simulink model "leaderAppl"  (R2022a)
settings: Solver=ode1  StartTime=0.0  StopTime=Inf  FixedStep=0.001  RelTol=1e-3
PreLoadFcn:
  | % 64-bit float
  | TurnSignalLeverValue = Simulink.Parameter;
  | TurnSignalLeverValue.StorageClass = 'ExportedGlobal';
  | TurnSignalLeverValue.DataType = 'double'
  | TurnSignalLeverValue.Value = 0.0
  | 
  | % 64-bit float
  | WarningLightSwitchValue= Simulink.Parameter;
  | WarningLightSwitchValue.StorageClass = 'ExportedGlobal';
  | WarningLightSwitchValue.DataType = 'double'
  | WarningLightSwitchValue.Value = 0.0
  | 
  | % 64-bit float
  | BatteryVoltageValue = Simulink.Parameter;
  | BatteryVoltageValue.StorageClass = 'ExportedGlobal';
  | BatteryVoltageValue.DataType = 'double'
  | BatteryVoltageValue.Value = 12.5
  | 
  | % 64-bit float
  | SyncValue = Simulink.Parameter;
  | SyncValue.StorageClass = 'ExportedGlobal';
  | SyncValue.DataType = 'double'
  | SyncValue.Value = 0.0
  | 
  | % 64-bit float
  | WarningLightIndicator = Simulink.Signal;
  | WarningLightIndicator.StorageClass = 'ExportedGlobal';
  | 
  | % 64-bit float
  | FrontLightEcuTurnSignalLeft = Simulink.Signal;
  | FrontLightEcuTurnSignalLeft.StorageClass = 'ExportedGlobal';
  | 
  | % 64-bit float
  | FrontLightEcuTurnSignalRight = Simulink.Signal;
  | FrontLightEcuTurnSignalRight.StorageClass = 'ExportedGlobal';
  | 
  | % 64-bit float
  | RearLightEcuTurnSignalLeft = Simulink.Signal;
  | RearLightEcuTurnSignalLeft.StorageClass = 'ExportedGlobal';
  | 
  | % 64-bit float
  | RearLightEcuTurnSignalRight = Simulink.Signal;
  | RearLightEcuTurnSignalRight.StorageClass = 'ExportedGlobal';
PostLoadFcn:
  | , if any(exist('dsrtsu_mdlpostloadfcn', 'file') ~= 0), dsrtsu_mdlpostloadfcn('Execute', bdroot); end,
  | 
  | % Begin Version: 1.0
  | if(3 == exist('DSWatchDog')), DSWatchDog('OpenModel', get_param(bdroot(gcs),'filename')); end; assignin('base', sprintf('DS_%s_STATE', upper(bdroot(gcs))), 0);
  | % End Version: 1.0
InitFcn:
  | , if any(exist('rtifpga_mdlclblib', 'file') ~= 0), rtifpga_mdlclblib('Init', bdroot); end,
  | , if any(exist('dsmpb_private', 'file') ~= 0), dsmpb_private('dsmpb_mdlclblib', 'Init', bdroot); end,
StartFcn:
  | % Begin Version: 1.0
  | if(3 == exist('DSWatchDog')), DSWatchDog('StartModel', get_param(bdroot(gcs),'filename')); end; assignin('base', sprintf('DS_%s_STATE', upper(bdroot(gcs))), 2);
  | % End Version: 1.0
StopFcn:
  | % Begin Version: 1.0
  | if(3 == exist('DSWatchDog')), DSWatchDog('StopModel', get_param(bdroot(gcs),'filename')); end; assignin('base', sprintf('DS_%s_STATE', upper(bdroot(gcs))), 0);
  | % End Version: 1.0
libraries: simulink x2, simulink_extras x2
PreSaveFcn:
  | , if any(exist('dsmpb_private', 'file') ~= 0), dsmpb_private('dsmpb_mdlclblib', 'PreSave', bdroot); end,
  | 
  | % Begin Version: 1.0
  | OldName = get_param(bdroot(gcs), 'Tag'); NewName = get_param(bdroot(gcs), 'filename'); if (~strcmp(OldName, NewName)), if(3 == exist('DSWatchDog')), DSWatchDog('CloseModel', OldName); DSWatchDog('OpenModel', NewName); end; set_param(bdroot(gcs), 'Tag', NewName); end; try, evalin('base', 'clear OldName NewName'); catch, disp('Error during execution of PreSaveFcn callback'); end;
  | % End Version: 1.0
PostSaveFcn:
  | % Begin Version: 1.0
  | if(3 == exist('DSWatchDog')), DSWatchDog('SaveModel', get_param(bdroot(gcs),'filename')); end;
  | % End Version: 1.0
CloseFcn:
  | , if any(exist('dsmpb_private', 'file') ~= 0), dsmpb_private('dsmpb_mdlclblib', 'Close', bdroot); end,
  | % Begin Version: 1.0
  | if(3 == exist('DSWatchDog')), DSWatchDog('CloseModel', get_param(bdroot(gcs),'filename')); end; try, DS_STATE_NAME = sprintf('DS_%s_STATE', upper(bdroot(gcs))); evalin('base', 'clear(DS_STATE_NAME)'); evalin('base', 'clear DS_STATE_NAME'); catch, disp('Error during execution of CloseFcn callback'); end;
  | % End Version: 1.0
settings Model: Tag=C:\Users\dSPACE GmbH\Documents\dSPACE\Real-Time Testing\2023-B\SampleExperiments\TurnSignal_VEOSVECUMC\TurnSignal_VEOSVECUMC\Models\masterAppl.slx  RTICANMMDATA=struct('GeneralSetupData',struct('modelroot',['C:\Users\Admin\Documents\dSPACE\Real-Time Testing\3.2\SampleExperiments\TurnSignal_VEOSMC\Model'],'generalsettings',struct('filesettings',struct('destfolder',struct('Name','RTICANMM_FILES','Check',1),'buildfolder',struct('Name','.','Check',1),'AbsDestfolder',struct('Name',['C:\Users\Admin\Documents\dSPACE\Real-Time Testing\3.2\SampleExperiments\TurnSignal_VEOSMC\Model\RTICANMM_FILES']),'AbsBuildfolder',struct('Name',['C:\Users\Admin\Documents\dSPACE\Real-Time Testing\3.2\SampleExperiments\TurnSignal_VEOSMC\Model']))),'options',struct('addpaths',1,'rmpaths',1,'addtrcexclusion',logical(1),'cannavigator',struct('checkmonitoring',0),'show_usrtrc',0,'use_usrtrc',0),'advanced',struct('options',ones(1,100)),'MPSetup',{{}},'modelname','masterAppl','block','masterAppl'))  RTILINMMDATA=struct('GeneralSetupData',[])  DSRTSU_INTERNAL_RTI_VER=620  DSRTSU_INTERNAL_RTI_TYPE=rti1202  DSRTSU_INTERNAL_RTIFPGA=200  DSRTSU_INTERNAL_RTISTBM_VER=23.2  ModifiedByFormat=dSPACE GmbH  ExtModeTrigMode=oneshot  ExtModeArmWhenConnect=off  Creator=dSPACE GmbH  LastModifiedBy=dSPACE GmbH
settings SolverCC: AlgebraicLoopSolver=TrustRegion
settings DataIOCC: LimitDataPoints=on  SaveFormat=Structure  SignalLoggingSaveFormat=ModelDataLogs  ReturnWorkspaceOutputs=off
settings OptimizationCC: BlockReduction=off  ConditionallyExecuteInputs=off  OptimizeBlockIOStorage=off  BufferReuse=off  GlobalBufferReuse=off  ExpressionFolding=off  ExpressionDepthLimit=2147483647  LocalBlockOutputs=off  InitFltsAndDblsToZero=on  LifeSpan=inf
settings DebuggingCC: SaveWithParameterizedLinksMsg=none  UnderspecifiedInitializationDetection=Classic  MergeDetectMultiDrivingBlocksExec=none  SignalResolutionControl=TryResolveAllWithWarning  MultiTaskDSMMsg=warning  MultiTaskCondExecSysMsg=none  MultiTaskRateTransMsg=warning  TasksWithSamePriorityMsg=none  FcnCallInpInsideContextMsg=warning  UnconnectedInputMsg=warning  UnconnectedOutputMsg=warning  UnconnectedLineMsg=warning  AllowSymbolicDim=off  StateNameClashWarn=warning  SFUnexpectedBacktrackingDiag=warning  SFNoUnconditionalDefaultTransitionDiag=warning  SFExecutionAtInitializationDiag=none  SFMachineParentedDataDiag=warning  ArithmeticOperatorsInVariantConditions=warning
settings HardwareCC: ProdBitPerLong=64  ProdLargestAtomicInteger=Integer  ProdWordSize=32  ProdHWDeviceType=Custom Processor->Custom  TargetIntDivRoundTo=Zero  TargetEndianess=LittleEndian  TargetHWDeviceType=Generic->Custom
settings ModelReferenceCC: PropagateSignalLabelsOutOfModel=off
settings SFSimCC: SimUseLocalCustomCode=off  CustomCodeUndefinedFunction=UseInterfaceOnly
settings RTWCC: Description=dSPACE Run-Time Target  SystemTargetFile=dsrt.tlc  GenCodeOnly=on  MakeCommand=make_dsrt  TemplateMakefile=dsrt_default_tmf  RTWVerbose=off  RTWUseLocalCustomCode=off
settings CodeAppCC: StateflowObjectComments=on
settings STFCustomTargetCC: ParMdlRefBuildCompliant=on  GRTInterface=off  SystemTargetFile=dsrt.tlc
settings GRTTargetCC: TargetLangStandard=C89/C90 (ANSI)  CompOptLevelCompliant=off  ConcurrentExecutionCompliant=off  CombineOutputUpdateFcns=off  MatFileLogging=off  CPPClassGenCompliant=off  UseToolchainInfoCompliant=off  GenerateASAP2=on
settings ConfigComp: CovMetricSettings=dw  CovSaveCumulativeToWorkspaceVar=on  CovSaveSingleToWorkspaceVar=on  CovExternalEMLEnable=off  CovSFcnEnable=off

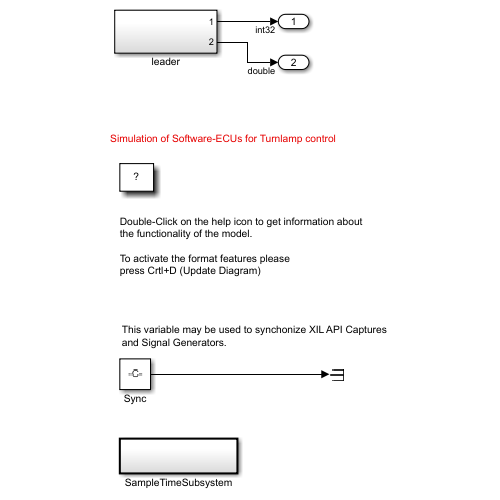
[thumbnail: Simulink's stored preview of the top-level diagram]
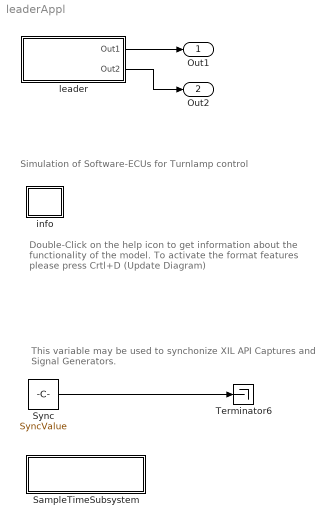
== system leaderAppl ==
  note: Simulation of Software-ECUs for Turnlamp control
  note: Double-Click on the help icon to get information about
      | the functionality of the model.
      |
      | To activate the format features please
      | press Crtl+D (Update Diagram)
  note: This variable may be used to synchonize XIL API Captures
      | and Signal Generators.
  SampleTimeSubsystem : Subsystem  TreatAsAtomicUnit=on  SystemSampleTime=0.01
  Sync : Constant  Value=SyncValue
  Terminator6 : Terminator
  info : Subsystem
      mask Display: disp('?')
  leader : Subsystem
  Out1 : Outport  OutDataTypeStr=int32  PortDimensions=1
  Out2 : Outport  Port=2  OutDataTypeStr=double  PortDimensions=1
  wires:
  leader/1(Out1) -> Out1/1
  leader/2(Out2) -> Out2/1
  Sync/1 -> Terminator6/1

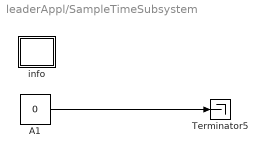
== system leaderAppl/SampleTimeSubsystem ==
  A1 : Constant  Value=0
  Terminator5 : Terminator
  info : Subsystem
      mask Display: disp('?')
  wires:
  A1/1 -> Terminator5/1

== system leaderAppl/info ==
  note: .
  note: This model simulates the behaviour of three ECUs for controlling TurnSignals,
      | dependent on a TurnSignalLever and a WarningLightSwitch
  note: Aim of this demo: to show possibilities of different ECU test procedures
  note: To control this model, use the corresponding ControlDesk experiment:
      | - Set TurnSignalLever to Left, Right or Off
      | - Switch WarningLight Switch to Off or On
      | - Change the Battery voltage: below a certain voltage level, some (simulated) malfunctions may occur
      |    - <= 7.2V, the ECUs will collapse completely
      |    - <= 8.2 V (dependent on voltage, more effect with lower voltage), simulated receiver in front and rear ECU become unstable,
      |      thus the timing of the generated TurnSignal will be disturbed

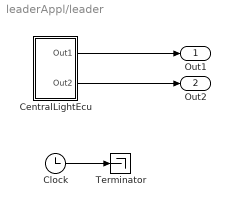
== system leaderAppl/leader ==
  CentralLightEcu : Subsystem
  Clock : Clock
  Terminator : Terminator
  Out1 : Outport
  Out2 : Outport  Port=2
  wires:
  CentralLightEcu/1(Out1) -> Out1/1
  CentralLightEcu/2(Out2) -> Out2/1
  Clock/1 -> Terminator/1

== system leaderAppl/SampleTimeSubsystem/info ==
  note: .
  note: This subsystems realizes a new sampling period for measurements. It is configured with a step size of 10 ms.

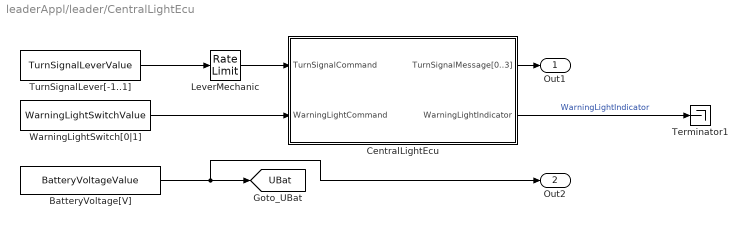
== system leaderAppl/leader/CentralLightEcu ==
  BatteryVoltage[V] : Constant  Value=BatteryVoltageValue
  CentralLightEcu : Subsystem
  LeverMechanic : RateLimiter  RisingSlewLimit=25  FallingSlewLimit=-25
  Terminator1 : Terminator
  TurnSignalLever[-1..1] : Constant  Value=TurnSignalLeverValue
  WarningLightSwitch[0|1] : Constant  Value=WarningLightSwitchValue
  Out1 : Outport
  Out2 : Outport  Port=2
  tag scope: UBat=global
  wires:
  CentralLightEcu/1(TurnSignalMessage[0..3]) -> Out1/1
  BatteryVoltage[V]/1 -> Out2/1, [UBat]
  CentralLightEcu/2(WarningLightIndicator) -> Terminator1/1  "WarningLightIndicator"
  WarningLightSwitch[0|1]/1 -> CentralLightEcu/2(WarningLightCommand)
  LeverMechanic/1 -> CentralLightEcu/1(TurnSignalCommand)
  TurnSignalLever[-1..1]/1 -> LeverMechanic/1

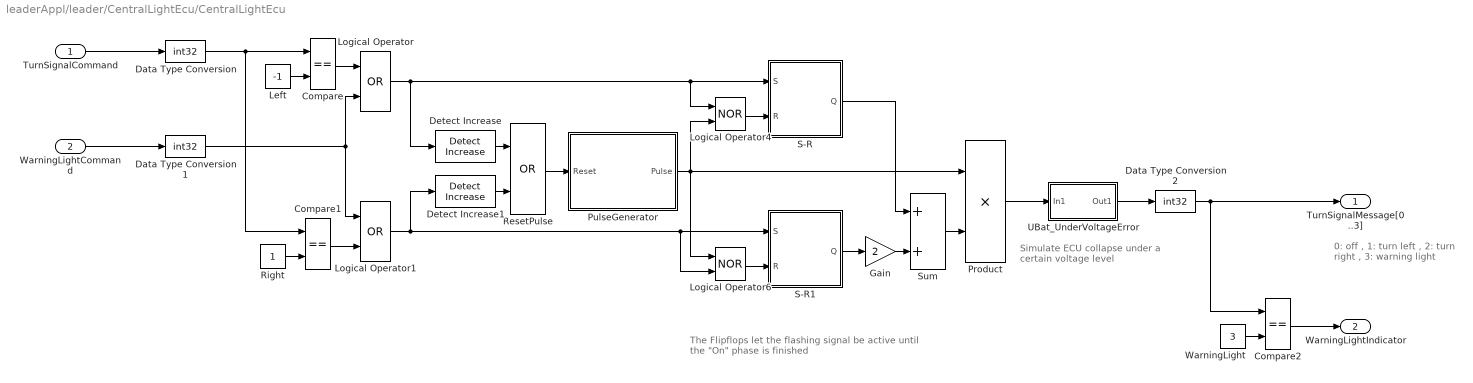
== system leaderAppl/leader/CentralLightEcu/CentralLightEcu ==
  note: The Flipflops let the flashing signal be active until
      | the "On" phase is finished
  note: Simulate ECU collapse
      | under a certain voltage level
  note: 0: off               ,
      | 1: turn left       ,
      | 2: turn right     ,
      | 3: warning light
  TurnSignalCommand : Inport
  WarningLightCommand : Inport  Port=2
  Compare : RelationalOperator  Operator===  OutDataTypeStr=uint(8)  ZeroCross=off
  Compare1 : RelationalOperator  Operator===  OutDataTypeStr=uint(8)  ZeroCross=off
  Compare2 : RelationalOperator  Operator===  OutDataTypeStr=uint(8)  ZeroCross=off
  Data Type Conversion : DataTypeConversion  OutDataTypeStr=int32  SaturateOnIntegerOverflow=off
  Data Type Conversion1 : DataTypeConversion  OutDataTypeStr=int32  SaturateOnIntegerOverflow=off
  Data Type Conversion2 : DataTypeConversion  OutDataTypeStr=int32  SaturateOnIntegerOverflow=off
  Detect Increase : simulink/Logic and Bit Operations/Detect Increase  vinit=0.0  OutDataTypeStr=boolean
  Detect Increase1 : simulink/Logic and Bit Operations/Detect Increase  vinit=0.0  OutDataTypeStr=boolean
  Gain : Gain  Gain=2
  Left : Constant  Value=-1  OutDataTypeStr=Inherit: Inherit via back propagation
  Logical Operator : Logic  Operator=OR  AllPortsSameDT=off  OutDataTypeStr=uint(8)
  Logical Operator1 : Logic  Operator=OR  AllPortsSameDT=off  OutDataTypeStr=uint(8)
  Logical Operator4 : Logic  Operator=NOR  AllPortsSameDT=off  OutDataTypeStr=uint(8)
  Logical Operator6 : Logic  Operator=NOR  AllPortsSameDT=off  OutDataTypeStr=uint(8)
  Product : Product  RndMeth=Zero
  PulseGenerator : Subsystem
  ResetPulse : Logic  Operator=OR  AllPortsSameDT=off  OutDataTypeStr=uint(8)
  Right : Constant  OutDataTypeStr=Inherit: Inherit via back propagation
  S-R : Subsystem
  S-R1 : Subsystem
  Sum : Sum
  UBat_UnderVoltageError : Subsystem
  WarningLight : Constant  Value=3  OutDataTypeStr=Inherit: Inherit via back propagation
  TurnSignalMessage[0..3] : Outport  OutDataTypeStr=int32
  WarningLightIndicator : Outport  Port=2
  wires:
  WarningLight/1 -> Compare2/2
  Right/1 -> Compare1/2
  Left/1 -> Compare/2
  Data Type Conversion2/1 -> Compare2/1, TurnSignalMessage[0..3]/1
  UBat_UnderVoltageError/1(Out1) -> Data Type Conversion2/1
  S-R/1(Q) -> Sum/1
  S-R1/1(Q) -> Gain/1
  Sum/1 -> Product/2
  PulseGenerator/1(Pulse) -> Product/1, Logical Operator6/1, Logical Operator4/2
  ResetPulse/1 -> PulseGenerator/1(Reset)
  Detect Increase1/1 -> ResetPulse/2
  Detect Increase/1 -> ResetPulse/1
  Logical Operator1/1 -> S-R1/1(S), Logical Operator6/2, Detect Increase1/1
  Logical Operator6/1 -> S-R1/2(R)
  Logical Operator4/1 -> S-R/2(R)
  Logical Operator/1 -> Detect Increase/1, S-R/1(S), Logical Operator4/1
  Compare2/1 -> WarningLightIndicator/1
  WarningLightCommand/1 -> Data Type Conversion1/1
  Product/1 -> UBat_UnderVoltageError/1(In1)
  TurnSignalCommand/1 -> Data Type Conversion/1
  Gain/1 -> Sum/2
  Compare1/1 -> Logical Operator1/2
  Data Type Conversion1/1 -> Logical Operator1/1, Logical Operator/2
  Compare/1 -> Logical Operator/1
  Data Type Conversion/1 -> Compare1/1, Compare/1

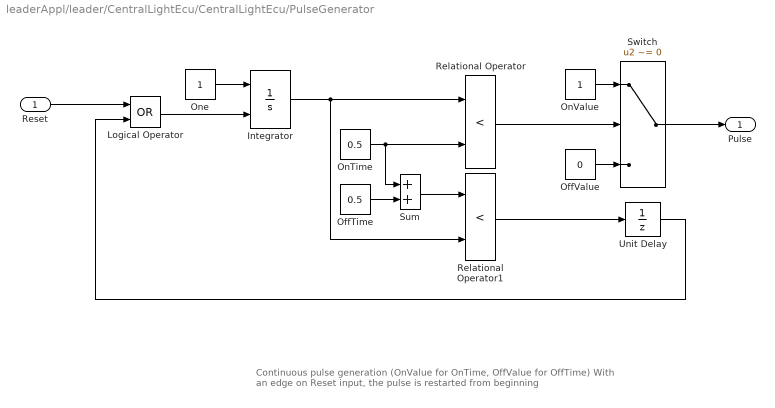
== system leaderAppl/leader/CentralLightEcu/CentralLightEcu/PulseGenerator ==
  note: Continuous pulse generation (OnValue for OnTime, OffValue for OffTime)
      | With an edge on Reset input, the pulse is restarted from beginning
  Reset : Inport
  Integrator : Integrator  ExternalReset=rising
  Logical Operator : Logic  Operator=OR  AllPortsSameDT=off  OutDataTypeStr=boolean
  OffTime : Constant  Value=0.5
  OffValue : Constant  Value=0
  OnTime : Constant  Value=0.5
  OnValue : Constant
  One : Constant
  Relational Operator : RelationalOperator  Operator=<  OutDataTypeStr=boolean  InputSameDT=off
  Relational Operator1 : RelationalOperator  Operator=<  OutDataTypeStr=boolean  InputSameDT=off
  Sum : Sum
  Switch : Switch  Criteria=u2 ~= 0  SaturateOnIntegerOverflow=off  InputSameDT=off
  Unit Delay : UnitDelay  SampleTime=-1  HasFrameUpgradeWarning=on
  Pulse : Outport
  wires:
  Unit Delay/1 -> Logical Operator/2
  Reset/1 -> Logical Operator/1
  Logical Operator/1 -> Integrator/2
  Relational Operator1/1 -> Unit Delay/1
  Sum/1 -> Relational Operator1/1
  OffTime/1 -> Sum/2
  One/1 -> Integrator/1
  OffValue/1 -> Switch/3
  OnValue/1 -> Switch/1
  Relational Operator/1 -> Switch/2
  OnTime/1 -> Sum/1, Relational Operator/2
  Integrator/1 -> Relational Operator1/2, Relational Operator/1
  Switch/1 -> Pulse/1

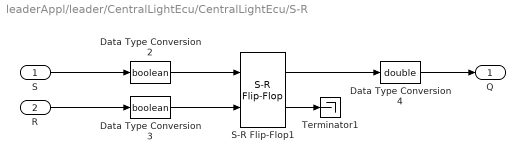
== system leaderAppl/leader/CentralLightEcu/CentralLightEcu/S-R ==
  S : Inport
  R : Inport  Port=2
  Data Type Conversion2 : DataTypeConversion  OutDataTypeStr=boolean  SaturateOnIntegerOverflow=off
  Data Type Conversion3 : DataTypeConversion  OutDataTypeStr=boolean  SaturateOnIntegerOverflow=off
  Data Type Conversion4 : DataTypeConversion  OutDataTypeStr=double  SaturateOnIntegerOverflow=off
  S-R Flip-Flop1 : simulink_extras/Flip Flops/S-R Flip-Flop  initial_condition=0
  Terminator1 : Terminator
  Q : Outport
  wires:
  S-R Flip-Flop1/2 -> Terminator1/1
  Data Type Conversion2/1 -> S-R Flip-Flop1/1
  Data Type Conversion3/1 -> S-R Flip-Flop1/2
  S-R Flip-Flop1/1 -> Data Type Conversion4/1
  S/1 -> Data Type Conversion2/1
  Data Type Conversion4/1 -> Q/1
  R/1 -> Data Type Conversion3/1

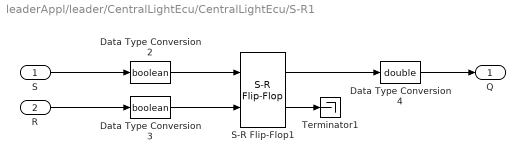
== system leaderAppl/leader/CentralLightEcu/CentralLightEcu/S-R1 ==
  S : Inport
  R : Inport  Port=2
  Data Type Conversion2 : DataTypeConversion  OutDataTypeStr=boolean  SaturateOnIntegerOverflow=off
  Data Type Conversion3 : DataTypeConversion  OutDataTypeStr=boolean  SaturateOnIntegerOverflow=off
  Data Type Conversion4 : DataTypeConversion  OutDataTypeStr=double  SaturateOnIntegerOverflow=off
  S-R Flip-Flop1 : simulink_extras/Flip Flops/S-R Flip-Flop  initial_condition=0
  Terminator1 : Terminator
  Q : Outport
  wires:
  R/1 -> Data Type Conversion3/1
  Data Type Conversion4/1 -> Q/1
  S/1 -> Data Type Conversion2/1
  S-R Flip-Flop1/1 -> Data Type Conversion4/1
  Data Type Conversion3/1 -> S-R Flip-Flop1/2
  Data Type Conversion2/1 -> S-R Flip-Flop1/1
  S-R Flip-Flop1/2 -> Terminator1/1

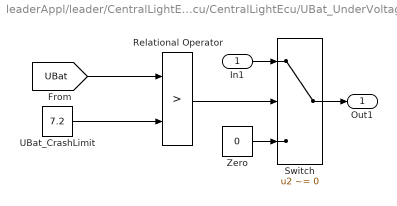
== system leaderAppl/leader/CentralLightEcu/CentralLightEcu/UBat_UnderVoltageError ==
  In1 : Inport
  Relational Operator : RelationalOperator  Operator=>  OutDataTypeStr=boolean  InputSameDT=off
  Switch : Switch  Criteria=u2 ~= 0  SaturateOnIntegerOverflow=off  InputSameDT=off
  UBat_CrashLimit : Constant  Value=7.2
  Zero : Constant  Value=0
  Out1 : Outport
  wires:
  Switch/1 -> Out1/1
  In1/1 -> Switch/1
  Zero/1 -> Switch/3
  Relational Operator/1 -> Switch/2
  [UBat] -> Relational Operator/1
  UBat_CrashLimit/1 -> Relational Operator/2
